simulink model "Statechart_Test_4_Ref"  (R2016b)
settings: Solver=VariableStepAuto  StartTime=0.0  StopTime=10.0  RelTol=1e-3  EnableMultiTasking=on
settings Model: Creator=Rose  LastModifiedBy=Rose
settings OptimizationCC: LifeSpan=inf
settings DebuggingCC: SFUnexpectedBacktrackingDiag=warning  SFNoUnconditionalDefaultTransitionDiag=warning  SFExecutionAtInitializationDiag=none
settings GRTTargetCC: TargetLangStandard=C89/C90 (ANSI)
settings ConfigComp: CovMetricSettings=dw  CovHtmlReporting=on  CovSaveCumulativeToWorkspaceVar=on  CovSaveSingleToWorkspaceVar=on  CovExternalEMLEnable=off

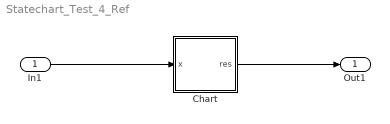
== system Statechart_Test_4_Ref ==
  In1 : Inport
  Chart : Stateflow chart  TreatAsAtomicUnit=on
  Out1 : Outport
  wires:
  In1/1 -> Chart/1(x)
  Chart/1(res) -> Out1/1

== stateflow chart Statechart_Test_4_Ref/Chart ==
  state START
  state END
  state MULT
    entry: x := x - 1
    exit: res = res * x
  (default) -> START
  START -> END [order 1] : [x == 1 || x == 0] /{ res = 1}
  MULT -> MULT [order 1] : [x > 1]
  START -> MULT [order 2] : [x > 1] / { res = x}
  MULT -> END [order 2] : [x == 1]
  data: x input; res output; y local
